simulink model "AtmLastNull"  (R2015a)
settings: configuration reference "SIMULATION_CONFIGURATION" (kept outside this file)
settings Model: CovSFcnEnable=off  Creator=moritz  LastModifiedBy=moritz
settings ConfigSetRef: SourceLocation=Base Workspace

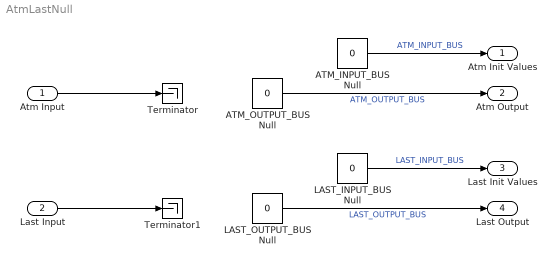
== system AtmLastNull ==
  Atm Input : Inport  OutDataTypeStr=Bus: ATM_INPUT_BUS  BusOutputAsStruct=on
  Last Input : Inport  Port=2  OutDataTypeStr=Bus: LAST_INPUT_BUS  BusOutputAsStruct=on
  ATM_INPUT_BUS Null : Constant  Value=0  OutDataTypeStr=Bus: ATM_INPUT_BUS  SampleTime=0
  ATM_OUTPUT_BUS Null : Constant  Value=0  OutDataTypeStr=Bus: ATM_OUTPUT_BUS  SampleTime=0
  LAST_INPUT_BUS Null : Constant  Value=0  OutDataTypeStr=Bus: LAST_INPUT_BUS  SampleTime=0
  LAST_OUTPUT_BUS Null : Constant  Value=0  OutDataTypeStr=Bus: LAST_OUTPUT_BUS  SampleTime=0
  Terminator : Terminator
  Terminator1 : Terminator
  Atm Init Values : Outport  OutDataTypeStr=Bus: ATM_INPUT_BUS  BusOutputAsStruct=on
  Atm Output : Outport  Port=2  OutDataTypeStr=Bus: ATM_OUTPUT_BUS  BusOutputAsStruct=on
  Last Init Values : Outport  Port=3  OutDataTypeStr=Bus: LAST_INPUT_BUS  BusOutputAsStruct=on
  Last Output : Outport  Port=4  OutDataTypeStr=Bus: LAST_OUTPUT_BUS  BusOutputAsStruct=on
  wires:
  ATM_OUTPUT_BUS Null/1 -> Atm Output/1  "ATM_OUTPUT_BUS"
  LAST_OUTPUT_BUS Null/1 -> Last Output/1  "LAST_OUTPUT_BUS"
  ATM_INPUT_BUS Null/1 -> Atm Init Values/1  "ATM_INPUT_BUS"
  LAST_INPUT_BUS Null/1 -> Last Init Values/1  "LAST_INPUT_BUS"
  Atm Input/1 -> Terminator/1
  Last Input/1 -> Terminator1/1
